simulink model "dsm_3rd_order_ciff_10mhz_topology_model"  (R2024a)
settings: Solver=FixedStepDiscrete  StartTime=0.0  StopTime=0.0008191  FixedStep=1e-07  RelTol=1e-3
model workspace (MAT data in the model file):
  A_dsm = [1  0  0; 1  1  -0.00577183233491; 0  1  1]
  B_dsm = [1  -1; 0  0; 0  0]
  C_dsm = [2.3625162736 2.02236426159 0.59546113812]
  D_dsm = [1 0]
  Ts_dsm = 1e-07
  x0_dsm = [0; 0; 0]
undefined symbols (not defined in the file or in its folder): dsm_quantizer
settings Model: Creator=sli767  LastModifiedBy=sli767

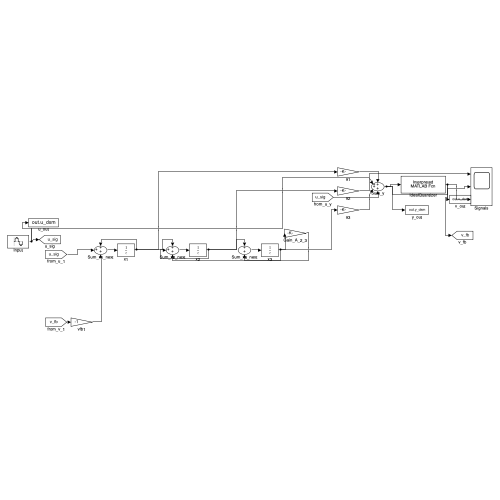
[thumbnail: Simulink's stored preview of the top-level diagram]
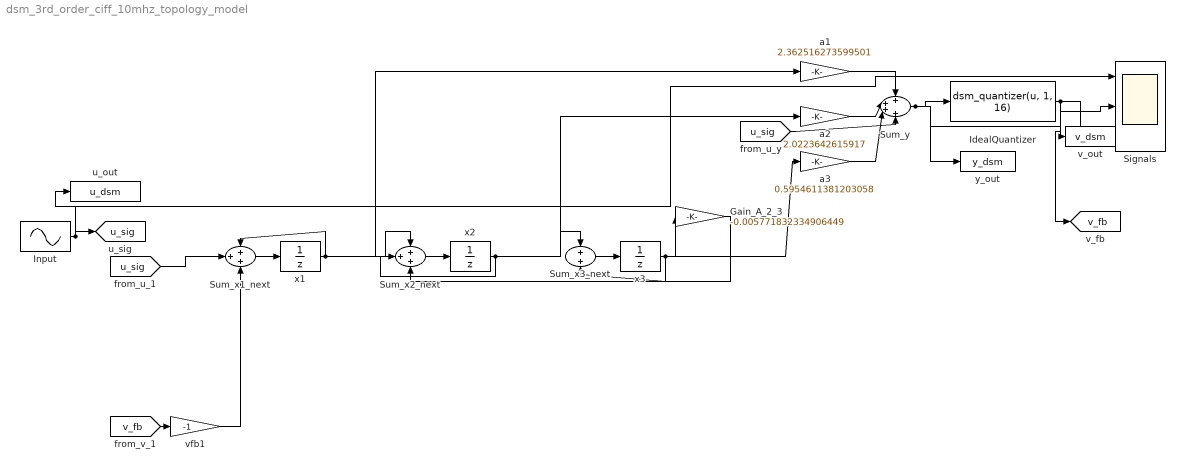
== system dsm_3rd_order_ciff_10mhz_topology_model ==
  Gain_A_2_3 : Gain  Gain=-0.005771832334906449
  IdealQuantizer : MATLABFcn  MATLABFcn=dsm_quantizer(u, 1, 16)
  Input : Sin  Amplitude=0.5  Frequency=368155.3890925539  SampleTime=1e-07
  Signals : Scope  NumInputPorts=3
  Sum_x1_next : Sum  Inputs=+++
  Sum_x2_next : Sum  Inputs=+++
  Sum_x3_next : Sum
  Sum_y : Sum  Inputs=++++
  a1 : Gain  Gain=2.362516273599501
  a2 : Gain  Gain=2.0223642615917
  a3 : Gain  Gain=0.5954611381203058
  u_out : ToWorkspace  VariableName=u_dsm  SampleTime=-1
  v_out : ToWorkspace  VariableName=v_dsm  SampleTime=-1
  vfb1 : Gain  Gain=-1
  x1 : UnitDelay  InitialCondition=x0_dsm(1)  SampleTime=Ts_dsm  HasFrameUpgradeWarning=on
  x2 : UnitDelay  InitialCondition=x0_dsm(2)  SampleTime=Ts_dsm  HasFrameUpgradeWarning=on
  x3 : UnitDelay  InitialCondition=x0_dsm(3)  SampleTime=Ts_dsm  HasFrameUpgradeWarning=on
  y_out : ToWorkspace  VariableName=y_dsm  SampleTime=-1
  tag scope: u_sig=global, v_fb=global
  wires:
  Input/1 -> [u_sig], u_out/1, Signals/1
  Sum_x1_next/1 -> x1/1
  Sum_x2_next/1 -> x2/1
  Sum_x3_next/1 -> x3/1
  x1/1 -> Sum_x1_next/1, Sum_x2_next/1, a1/1
  [u_sig] -> Sum_x1_next/2
  [v_fb] -> vfb1/1
  vfb1/1 -> Sum_x1_next/3
  x2/1 -> Sum_x2_next/2, Sum_x3_next/1, a2/1
  x3/1 -> Gain_A_2_3/1, Sum_x3_next/2, a3/1
  Gain_A_2_3/1 -> Sum_x2_next/3
  a1/1 -> Sum_y/1
  a2/1 -> Sum_y/2
  a3/1 -> Sum_y/3
  [u_sig] -> Sum_y/4
  Sum_y/1 -> IdealQuantizer/1, y_out/1, Signals/2
  IdealQuantizer/1 -> [v_fb], v_out/1, Signals/3
